simulink model "SOC"  (R2021a)
settings: Solver=VariableStepAuto  StartTime=0.0  StopTime=1180  RelTol=1e-3
undefined symbols (not defined in the file or in its folder): C1_LUT, Capacity_LUT, cell_area, cell_Cp_heat, cell_mass, Em_LUT, h_conv, R0_LUT, R1_LUT, SOC_LUT, T_init, Temperature_LUT
settings Model: Creator=SAHIL  LastModifiedBy=SAHIL

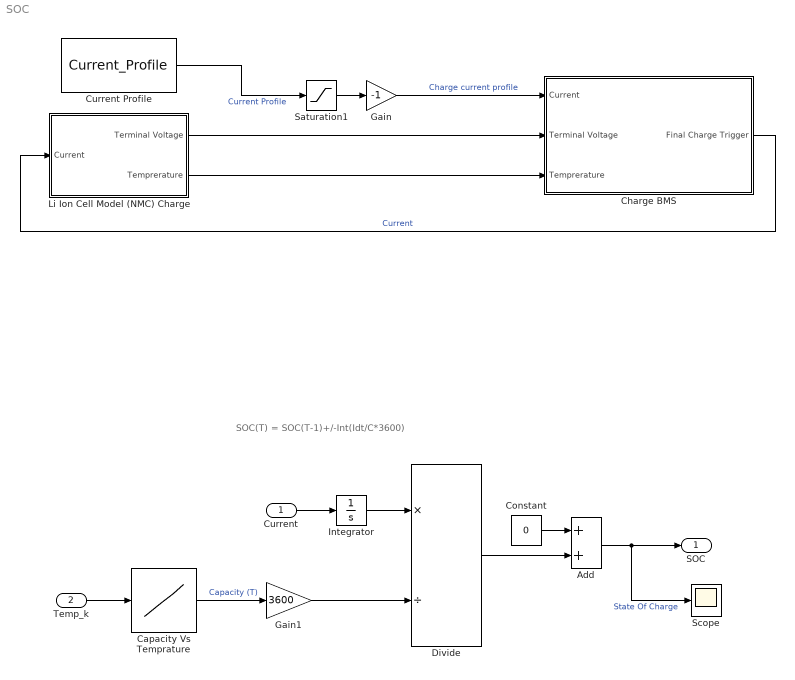
== system SOC ==
  note: SOC(T) = SOC(T-1)+/-Int(Idt/C*3600)
  Current : Inport
  Temp_k : Inport  Port=2
  Add : Sum
  Capacity Vs Temprature : Lookup_n-D  NumberOfTableDimensions=1  BreakpointsForDimension1=Temperature_LUT  Table=Capacity_LUT  InternalRulePriority=Speed  RndMeth=Simplest  InputSameDT=on
  Charge BMS : Subsystem
  Constant : Constant  Value=0
  Current Profile : FromWorkspace  VariableName=Current_Profile
  Divide : Product  Inputs=*/
  Gain : Gain  Gain=-1
  Gain1 : Gain  Gain=3600
  Integrator : Integrator
  Li Ion Cell Model (NMC) Charge : Subsystem
  Saturation1 : Saturate  UpperLimit=0  LowerLimit=-inf
  Scope : Scope
  SOC : Outport
  wires:
  Gain/1 -> Charge BMS/1(Current)  "Charge current profile"
  Li Ion Cell Model (NMC) Charge/2(Temprerature) -> Charge BMS/3(Temprerature)
  Saturation1/1 -> Gain/1
  Current Profile/1 -> Saturation1/1  "Current Profile"
  Li Ion Cell Model (NMC) Charge/1(Terminal Voltage) -> Charge BMS/2(Terminal Voltage)
  Add/1 -> Scope/1, SOC/1  "State Of Charge"
  Charge BMS/1(Final Charge Trigger) -> Li Ion Cell Model (NMC) Charge/1(Current)  "Current"
  Current/1 -> Integrator/1
  Gain1/1 -> Divide/2
  Constant/1 -> Add/1
  Divide/1 -> Add/2
  Capacity Vs Temprature/1 -> Gain1/1  "Capacity (T)"
  Temp_k/1 -> Capacity Vs Temprature/1
  Integrator/1 -> Divide/1

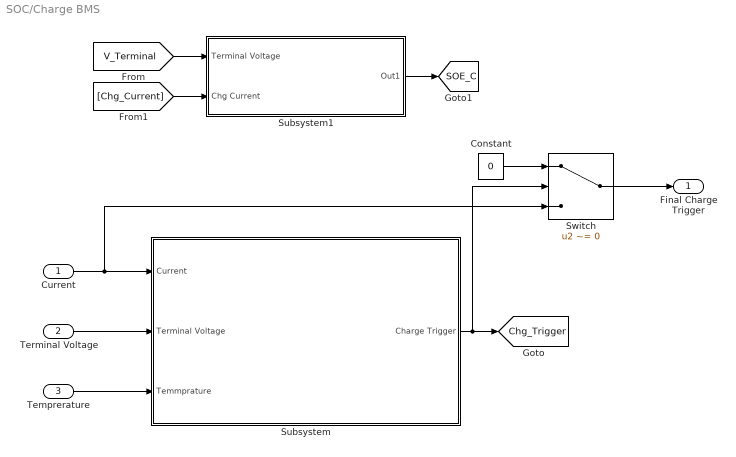
== system SOC/Charge BMS ==
  Current : Inport
  Terminal Voltage : Inport  Port=2
  Temprerature : Inport  Port=3
  Constant : Constant  Value=0
  Subsystem : Subsystem
  Subsystem1 : Subsystem
  Switch : Switch  Criteria=u2 ~= 0
  Final Charge Trigger : Outport
  tag scope: Chg_Trigger=global, SOE_C=global
  wires:
  Current/1 -> Switch/3, Subsystem/1(Current)
  Terminal Voltage/1 -> Subsystem/2(Terminal Voltage)
  Temprerature/1 -> Subsystem/3(Temmprature)
  Subsystem/1(Charge Trigger) -> Switch/2, [Chg_Trigger]
  Constant/1 -> Switch/1
  Switch/1 -> Final Charge Trigger/1
  Subsystem1/1(Out1) -> [SOE_C]
  [Chg_Current] -> Subsystem1/2(Chg Current)
  [V_Terminal] -> Subsystem1/1(Terminal Voltage)

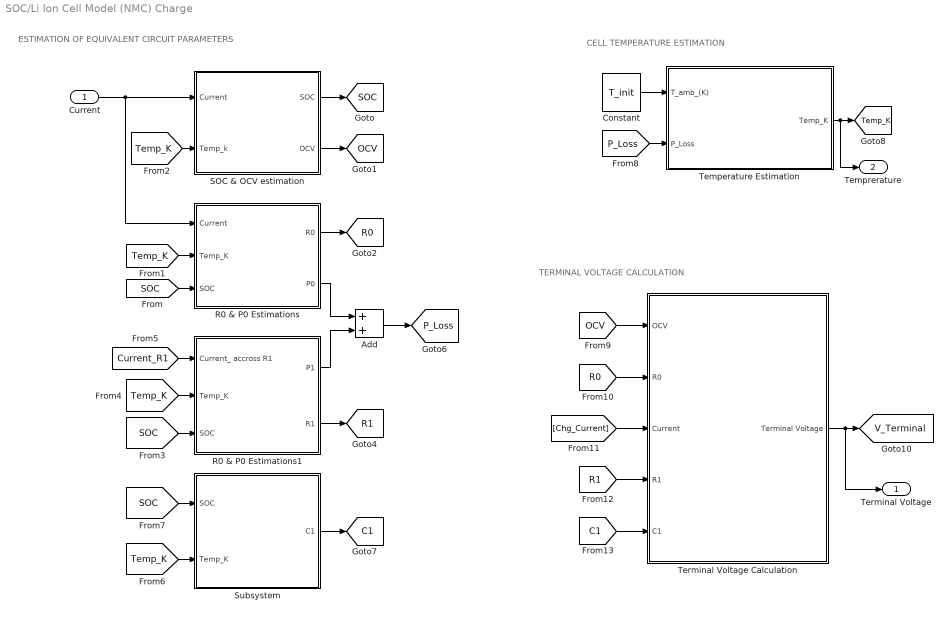
== system SOC/Li Ion Cell Model (NMC) Charge ==
  note: ESTIMATION OF EQUIVALENT CIRCUIT PARAMETERS
  note: CELL TEMPERATURE ESTIMATION
  note: TERMINAL VOLTAGE CALCULATION
  Current : Inport
  Add : Sum
  Constant : Constant  Value=T_init
  R0 & P0 Estimations : Subsystem
  R0 & P0 Estimations1 : Subsystem
  SOC & OCV estimation : Subsystem
  Subsystem : Subsystem
  Temperature Estimation : Subsystem
  Terminal Voltage Calculation : Subsystem
  Terminal Voltage : Outport
  Temprerature : Outport  Port=2
  tag scope: C1=global, OCV=global, P_Loss=global, R0=global, R1=global, SOC=global, Temp_K=global, V_Terminal=global
  wires:
  Terminal Voltage Calculation/1(Terminal Voltage) -> Terminal Voltage/1, [V_Terminal]
  [C1] -> Terminal Voltage Calculation/5(C1)
  [R1] -> Terminal Voltage Calculation/4(R1)
  [Chg_Current] -> Terminal Voltage Calculation/3(Current)
  [R0] -> Terminal Voltage Calculation/2(R0)
  [OCV] -> Terminal Voltage Calculation/1(OCV)
  [P_Loss] -> Temperature Estimation/2(P_Loss)
  Constant/1 -> Temperature Estimation/1(T_amb_(K))
  Temperature Estimation/1(Temp_K) -> Temprerature/1, [Temp_K]
  Subsystem/1(C1) -> [C1]
  R0 & P0 Estimations1/2(R1) -> [R1]
  Add/1 -> [P_Loss]
  R0 & P0 Estimations1/1(P1) -> Add/2
  [Current_R1] -> R0 & P0 Estimations1/1(Current_ accross R1)
  [Temp_K] -> R0 & P0 Estimations1/2(Temp_K)
  [SOC] -> R0 & P0 Estimations1/3(SOC)
  R0 & P0 Estimations/2(P0) -> Add/1
  R0 & P0 Estimations/1(R0) -> [R0]
  [Temp_K] -> R0 & P0 Estimations/2(Temp_K)
  [SOC] -> R0 & P0 Estimations/3(SOC)
  SOC & OCV estimation/2(OCV) -> [OCV]
  SOC & OCV estimation/1(SOC) -> [SOC]
  [Temp_K] -> SOC & OCV estimation/2(Temp_k)
  Current/1 -> SOC & OCV estimation/1(Current), R0 & P0 Estimations/1(Current)
  [SOC] -> Subsystem/1(SOC)
  [Temp_K] -> Subsystem/2(Temp_K)

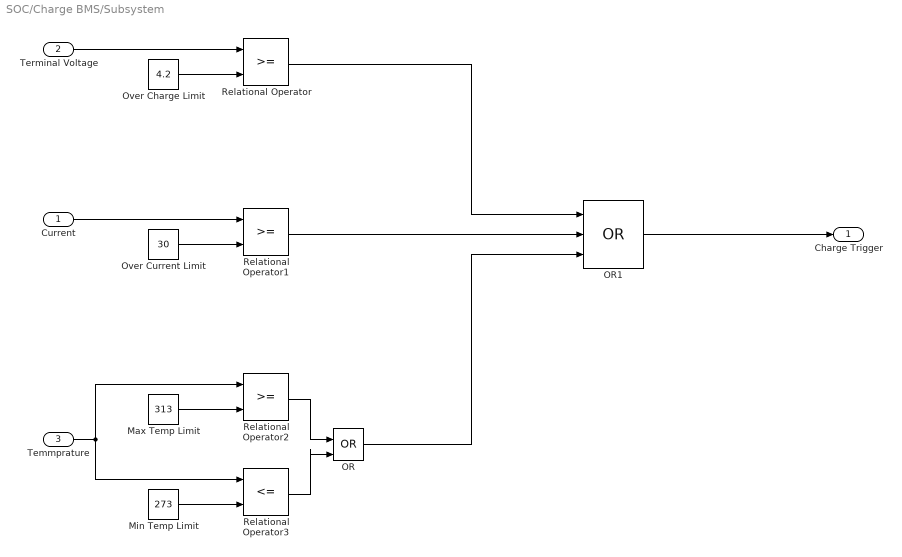
== system SOC/Charge BMS/Subsystem ==
  Current : Inport
  Terminal Voltage : Inport  Port=2
  Temmprature : Inport  Port=3
  Max Temp Limit : Constant  Value=313
  Min Temp Limit : Constant  Value=273
  OR : Logic  Operator=OR  IconShape=distinctive  AllPortsSameDT=off  OutDataTypeStr=boolean
  OR1 : Logic  Operator=OR  Inputs=3  IconShape=distinctive  AllPortsSameDT=off  OutDataTypeStr=boolean
  Over Charge Limit : Constant  Value=4.2
  Over Current Limit : Constant  Value=30
  Relational Operator : RelationalOperator  OutDataTypeStr=boolean  RndMeth=Simplest
  Relational Operator1 : RelationalOperator  OutDataTypeStr=boolean  RndMeth=Simplest
  Relational Operator2 : RelationalOperator  OutDataTypeStr=boolean  RndMeth=Simplest
  Relational Operator3 : RelationalOperator  Operator=<=  OutDataTypeStr=boolean  RndMeth=Simplest
  Charge Trigger : Outport
  wires:
  Min Temp Limit/1 -> Relational Operator3/2
  Relational Operator3/1 -> OR/2
  Relational Operator/1 -> OR1/1
  OR/1 -> OR1/3
  OR1/1 -> Charge Trigger/1
  Over Current Limit/1 -> Relational Operator1/2
  Relational Operator2/1 -> OR/1
  Max Temp Limit/1 -> Relational Operator2/2
  Over Charge Limit/1 -> Relational Operator/2
  Relational Operator1/1 -> OR1/2
  Terminal Voltage/1 -> Relational Operator/1
  Temmprature/1 -> Relational Operator3/1, Relational Operator2/1
  Current/1 -> Relational Operator1/1

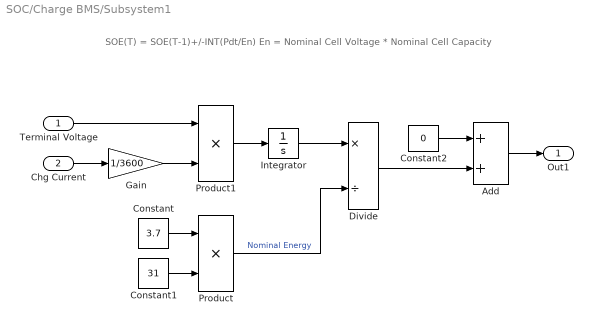
== system SOC/Charge BMS/Subsystem1 ==
  note: SOE(T) = SOE(T-1)+/-INT(Pdt/En)
      |
      | En = Nominal Cell Voltage * Nominal Cell Capacity
  Terminal Voltage : Inport
  Chg Current : Inport  Port=2
  Add : Sum
  Constant : Constant  Value=3.7
  Constant1 : Constant  Value=31
  Constant2 : Constant  Value=0
  Divide : Product  Inputs=*/
  Gain : Gain  Gain=1/3600
  Integrator : Integrator
  Product : Product
  Product1 : Product
  Out1 : Outport
  wires:
  Constant/1 -> Product/1
  Constant1/1 -> Product/2
  Product/1 -> Divide/2  "Nominal Energy"
  Chg Current/1 -> Gain/1
  Gain/1 -> Product1/2
  Terminal Voltage/1 -> Product1/1
  Product1/1 -> Integrator/1
  Integrator/1 -> Divide/1
  Constant2/1 -> Add/1
  Divide/1 -> Add/2
  Add/1 -> Out1/1

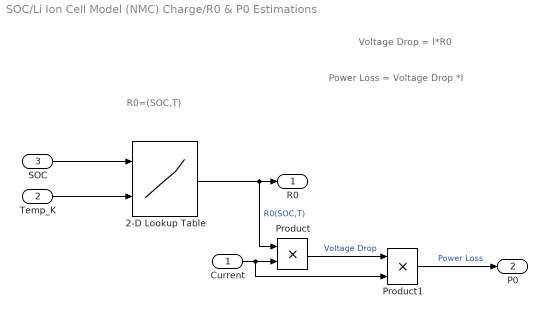
== system SOC/Li Ion Cell Model (NMC) Charge/R0 & P0 Estimations ==
  note: R0=(SOC,T)
  note: Voltage Drop = I*R0
  note: Power Loss = Voltage Drop *I
  Current : Inport
  Temp_K : Inport  Port=2
  SOC : Inport  Port=3
  2-D Lookup Table : Lookup_n-D  BreakpointsForDimension1=SOC_LUT  BreakpointsForDimension2=Temperature_LUT  Table=R0_LUT  InternalRulePriority=Speed  RndMeth=Simplest  InputSameDT=on
      settings: InputPortMap=u0,u1
  Product : Product
  Product1 : Product
  R0 : Outport
  P0 : Outport  Port=2
  wires:
  Product1/1 -> P0/1  "Power Loss"
  Product/1 -> Product1/1  "Voltage Drop"
  Current/1 -> Product/2, Product1/2
  2-D Lookup Table/1 -> R0/1, Product/1  "R0(SOC,T)"
  Temp_K/1 -> 2-D Lookup Table/2
  SOC/1 -> 2-D Lookup Table/1

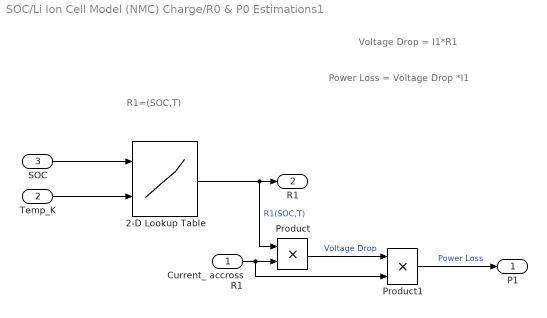
== system SOC/Li Ion Cell Model (NMC) Charge/R0 & P0 Estimations1 ==
  note: R1=(SOC,T)
  note: Voltage Drop = I1*R1
  note: Power Loss = Voltage Drop *I1
  Current_ accross R1 : Inport
  Temp_K : Inport  Port=2
  SOC : Inport  Port=3
  2-D Lookup Table : Lookup_n-D  BreakpointsForDimension1=SOC_LUT  BreakpointsForDimension2=Temperature_LUT  Table=R1_LUT  InternalRulePriority=Speed  RndMeth=Simplest  InputSameDT=on
      settings: InputPortMap=u0,u1
  Product : Product
  Product1 : Product
  P1 : Outport
  R1 : Outport  Port=2
  wires:
  Product1/1 -> P1/1  "Power Loss"
  Product/1 -> Product1/1  "Voltage Drop"
  Current_ accross R1/1 -> Product/2, Product1/2
  2-D Lookup Table/1 -> R1/1, Product/1  "R1(SOC,T)"
  Temp_K/1 -> 2-D Lookup Table/2
  SOC/1 -> 2-D Lookup Table/1

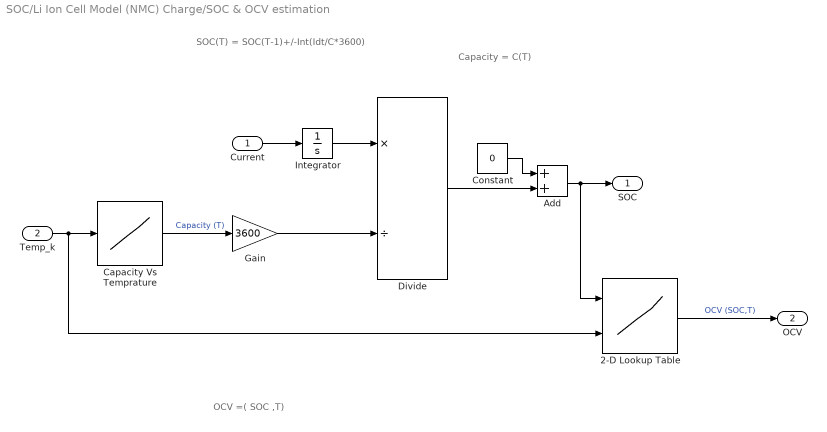
== system SOC/Li Ion Cell Model (NMC) Charge/SOC & OCV estimation ==
  note: SOC(T) = SOC(T-1)+/-Int(Idt/C*3600)
  note: Capacity = C(T)
  note: OCV =( SOC ,T)
  Current : Inport
  Temp_k : Inport  Port=2
  2-D Lookup Table : Lookup_n-D  BreakpointsForDimension1=SOC_LUT  BreakpointsForDimension2=Temperature_LUT  Table=Em_LUT  InternalRulePriority=Speed  RndMeth=Simplest  InputSameDT=on
      settings: InputPortMap=u0,u1
  Add : Sum
  Capacity Vs Temprature : Lookup_n-D  NumberOfTableDimensions=1  BreakpointsForDimension1=Temperature_LUT  Table=Capacity_LUT  InternalRulePriority=Speed  RndMeth=Simplest  InputSameDT=on
  Constant : Constant  Value=0
  Divide : Product  Inputs=*/
  Gain : Gain  Gain=3600
  Integrator : Integrator
  SOC : Outport
  OCV : Outport  Port=2
  wires:
  2-D Lookup Table/1 -> OCV/1  "OCV (SOC,T)"
  Add/1 -> SOC/1, 2-D Lookup Table/1
  Constant/1 -> Add/1
  Divide/1 -> Add/2
  Gain/1 -> Divide/2
  Integrator/1 -> Divide/1
  Current/1 -> Integrator/1
  Capacity Vs Temprature/1 -> Gain/1  "Capacity (T)"
  Temp_k/1 -> Capacity Vs Temprature/1, 2-D Lookup Table/2

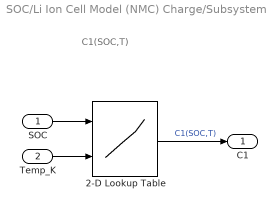
== system SOC/Li Ion Cell Model (NMC) Charge/Subsystem ==
  note: C1(SOC,T)
  SOC : Inport
  Temp_K : Inport  Port=2
  2-D Lookup Table : Lookup_n-D  BreakpointsForDimension1=SOC_LUT  BreakpointsForDimension2=Temperature_LUT  Table=C1_LUT  InternalRulePriority=Speed  RndMeth=Simplest  InputSameDT=on
      settings: InputPortMap=u0,u1
  C1 : Outport
  wires:
  2-D Lookup Table/1 -> C1/1  "C1(SOC,T)"
  Temp_K/1 -> 2-D Lookup Table/2
  SOC/1 -> 2-D Lookup Table/1

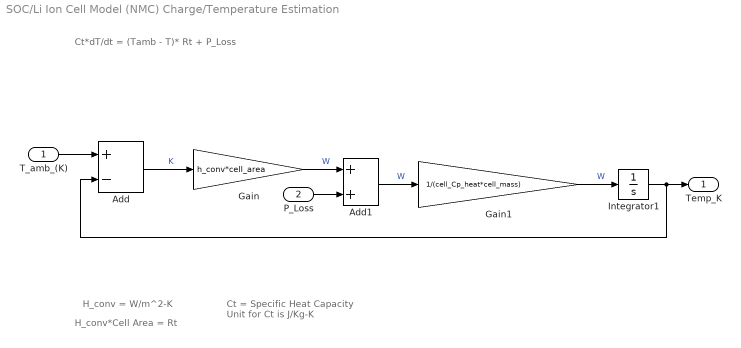
== system SOC/Li Ion Cell Model (NMC) Charge/Temperature Estimation ==
  note: Ct*dT/dt = (Tamb - T)* Rt + P_Loss
  note: H_conv = W/m^2-K
  note: H_conv*Cell Area = Rt
  note: Ct = Specific Heat Capacity
      | Unit for Ct is J/Kg-K
  T_amb_(K) : Inport
  P_Loss : Inport  Port=2
  Add : Sum  Inputs=+-
  Add1 : Sum
  Gain : Gain  Gain=h_conv*cell_area
  Gain1 : Gain  Gain=1/(cell_Cp_heat*cell_mass)
  Integrator1 : Integrator  InitialCondition=293.15
  Temp_K : Outport
  wires:
  Integrator1/1 -> Temp_K/1, Add/2
  Gain1/1 -> Integrator1/1  "W"
  Add1/1 -> Gain1/1  "W"
  P_Loss/1 -> Add1/2
  Gain/1 -> Add1/1  "W"
  Add/1 -> Gain/1  "K"
  T_amb_(K)/1 -> Add/1

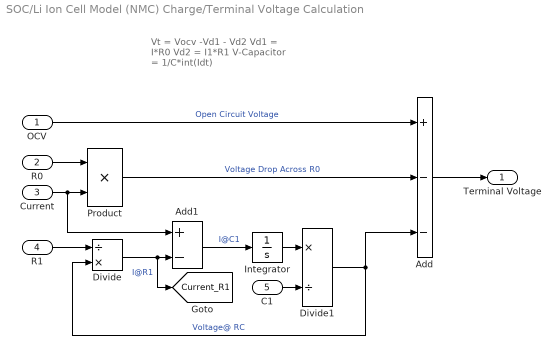
== system SOC/Li Ion Cell Model (NMC) Charge/Terminal Voltage Calculation ==
  note: Vt = Vocv -Vd1 - Vd2
      | Vd1 = I*R0
      | Vd2 = I1*R1
      | V-Capacitor = 1/C*int(Idt)
  OCV : Inport
  R0 : Inport  Port=2
  Current : Inport  Port=3
  R1 : Inport  Port=4
  C1 : Inport  Port=5
  Add : Sum  Inputs=+--
  Add1 : Sum  Inputs=+-
  Divide : Product  Inputs=/*
  Divide1 : Product  Inputs=*/
  Integrator : Integrator
  Product : Product
  Terminal Voltage : Outport
  tag scope: Current_R1=global
  wires:
  Divide1/1 -> Add/3, Divide/2  "Voltage@ RC"
  Integrator/1 -> Divide1/1
  C1/1 -> Divide1/2
  Add1/1 -> Integrator/1  "I@C1"
  Divide/1 -> [Current_R1], Add1/2  "I@R1"
  R1/1 -> Divide/1
  Product/1 -> Add/2  "Voltage Drop Across R0"
  Current/1 -> Product/2, Add1/1
  R0/1 -> Product/1
  Add/1 -> Terminal Voltage/1
  OCV/1 -> Add/1  "Open Circuit Voltage"
